simulink model "Quadcopter_nonlinear"  (R2020a)
settings: Solver=ode4  StartTime=0.0  StopTime=0.5  FixedStep=0.02  RelTol=1e-3
InitFcn:
  | QuadParameter
values from neighbouring files (symbols this model uses):
  d = 3.2e-6    (= 3.2e-06)    [QuadParameter.m]    (also in Scenario_III.mat)
  g = 9.81    [QuadParameter.m]
  init_I = data(1, :)    [load_data.m]
  init_II = data(1, :)    [load_data.m]
  init_III = data(1, :)    [load_data.m]
  init_IV = data(1, :)    [load_data.m]
  init_V = data(1, :)    [load_data.m]
  J_zz = 0.058510    (= 0.05851)    [QuadParameter.m]
  m3 = 1.693    [QuadParameter.m]
  miu_k = 0.002    [QuadParameter.m]
  Omega_I = Omega_data    [load_data.m]
  Omega_II = Omega_data    [load_data.m]
  Omega_III = Omega_data    [load_data.m]
  Omega_IV = Omega_data    [load_data.m]
  Omega_V = Omega_data    [load_data.m]
  r_z = 0.025    [QuadParameter.m]
undefined symbols (not defined in the file or in its folder): magnitude
settings Model: OrderedModelArguments=off  Creator=Ali  LastModifiedBy=Ali

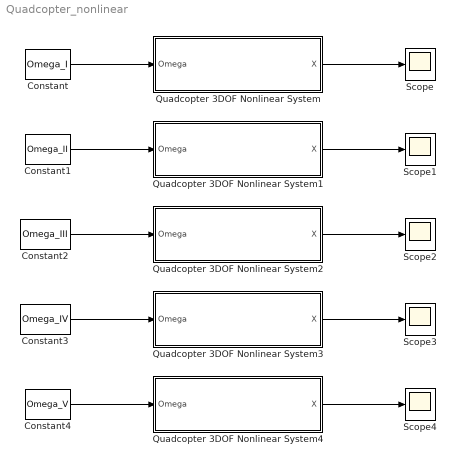
== system Quadcopter_nonlinear ==
  Constant : Constant  Value=Omega_I
  Constant1 : Constant  Value=Omega_II
  Constant2 : Constant  Value=Omega_III
  Constant3 : Constant  Value=Omega_IV
  Constant4 : Constant  Value=Omega_V
  Quadcopter 3DOF Nonlinear System : Subsystem  TreatAsAtomicUnit=on
  Quadcopter 3DOF Nonlinear System1 : Subsystem  TreatAsAtomicUnit=on
  Quadcopter 3DOF Nonlinear System2 : Subsystem  TreatAsAtomicUnit=on
  Quadcopter 3DOF Nonlinear System3 : Subsystem  TreatAsAtomicUnit=on
  Quadcopter 3DOF Nonlinear System4 : Subsystem  TreatAsAtomicUnit=on
  Scope{,1..4} (5 alike) : Scope
  wires:
  Quadcopter 3DOF Nonlinear System/1(X) -> Scope/1
  Constant/1 -> Quadcopter 3DOF Nonlinear System/1(Omega)
  Constant1/1 -> Quadcopter 3DOF Nonlinear System1/1(Omega)
  Quadcopter 3DOF Nonlinear System1/1(X) -> Scope1/1
  Constant2/1 -> Quadcopter 3DOF Nonlinear System2/1(Omega)
  Quadcopter 3DOF Nonlinear System2/1(X) -> Scope2/1
  Constant3/1 -> Quadcopter 3DOF Nonlinear System3/1(Omega)
  Quadcopter 3DOF Nonlinear System3/1(X) -> Scope3/1
  Constant4/1 -> Quadcopter 3DOF Nonlinear System4/1(Omega)
  Quadcopter 3DOF Nonlinear System4/1(X) -> Scope4/1

== system Quadcopter_nonlinear/Quadcopter 3DOF Nonlinear System ==
  Omega : Inport
  Integrator : Integrator  InitialCondition=init_I
  Quad System : Subsystem
  X : Outport
  wires:
  Integrator/1 -> Quad System/1(X), X/1  "X"
  Quad System/1(dot(X)) -> Integrator/1  "dot(X)"
  Omega/1 -> Quad System/2(Omega)

== system Quadcopter_nonlinear/Quadcopter 3DOF Nonlinear System1 ==
  Omega : Inport
  Integrator : Integrator  InitialCondition=init_II
  Quad System : Subsystem
  X : Outport
  wires:
  Integrator/1 -> Quad System/1(X), X/1  "X"
  Quad System/1(dot(X)) -> Integrator/1  "dot(X)"
  Omega/1 -> Quad System/2(Omega)

== system Quadcopter_nonlinear/Quadcopter 3DOF Nonlinear System2 ==
  Omega : Inport
  Integrator : Integrator  InitialCondition=init_III
  Quad System : Subsystem
  X : Outport
  wires:
  Integrator/1 -> Quad System/1(X), X/1  "X"
  Quad System/1(dot(X)) -> Integrator/1  "dot(X)"
  Omega/1 -> Quad System/2(Omega)

== system Quadcopter_nonlinear/Quadcopter 3DOF Nonlinear System3 ==
  Omega : Inport
  Integrator : Integrator  InitialCondition=init_IV
  Quad System : Subsystem
  X : Outport
  wires:
  Integrator/1 -> Quad System/1(X), X/1  "X"
  Quad System/1(dot(X)) -> Integrator/1  "dot(X)"
  Omega/1 -> Quad System/2(Omega)

== system Quadcopter_nonlinear/Quadcopter 3DOF Nonlinear System4 ==
  Omega : Inport
  Integrator : Integrator  InitialCondition=init_V
  Quad System : Subsystem
  X : Outport
  wires:
  Integrator/1 -> Quad System/1(X), X/1  "X"
  Quad System/1(dot(X)) -> Integrator/1  "dot(X)"
  Omega/1 -> Quad System/2(Omega)

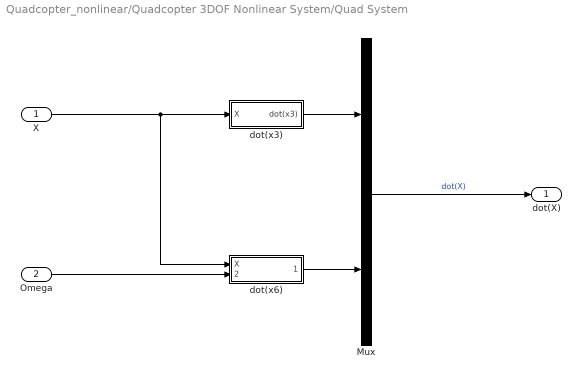
== system Quadcopter_nonlinear/Quadcopter 3DOF Nonlinear System/Quad System ==
  X : Inport
  Omega : Inport  Port=2
  Mux : Mux  Inputs=2
  dot(x3) : Subsystem
  dot(x6) : Subsystem
  dot(X) : Outport
  wires:
  Mux/1 -> dot(X)/1  "dot(X)"
  X/1 -> dot(x6)/1(X), dot(x3)/1(X)
  Omega/1 -> dot(x6)/2(Omega)
  dot(x3)/1(dot(x3)) -> Mux/1
  dot(x6)/1(dot(x6)) -> Mux/2

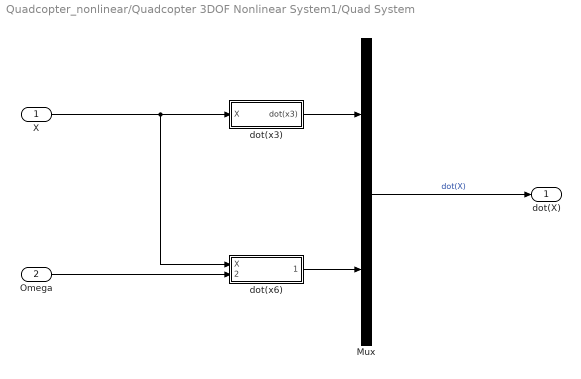
== system Quadcopter_nonlinear/Quadcopter 3DOF Nonlinear System1/Quad System ==
  X : Inport
  Omega : Inport  Port=2
  Mux : Mux  Inputs=2
  dot(x3) : Subsystem
  dot(x6) : Subsystem
  dot(X) : Outport
  wires:
  Mux/1 -> dot(X)/1  "dot(X)"
  X/1 -> dot(x6)/1(X), dot(x3)/1(X)
  Omega/1 -> dot(x6)/2(Omega)
  dot(x3)/1(dot(x3)) -> Mux/1
  dot(x6)/1(dot(x6)) -> Mux/2

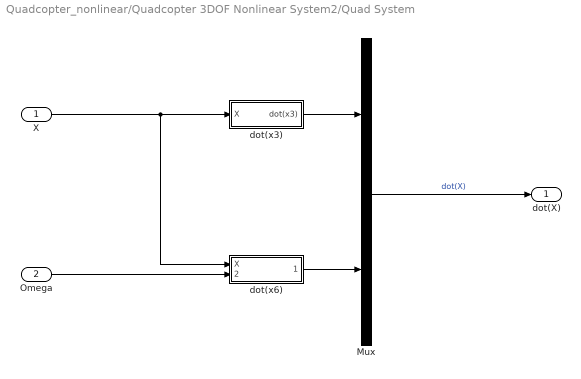
== system Quadcopter_nonlinear/Quadcopter 3DOF Nonlinear System2/Quad System ==
  X : Inport
  Omega : Inport  Port=2
  Mux : Mux  Inputs=2
  dot(x3) : Subsystem
  dot(x6) : Subsystem
  dot(X) : Outport
  wires:
  Mux/1 -> dot(X)/1  "dot(X)"
  X/1 -> dot(x6)/1(X), dot(x3)/1(X)
  Omega/1 -> dot(x6)/2(Omega)
  dot(x3)/1(dot(x3)) -> Mux/1
  dot(x6)/1(dot(x6)) -> Mux/2

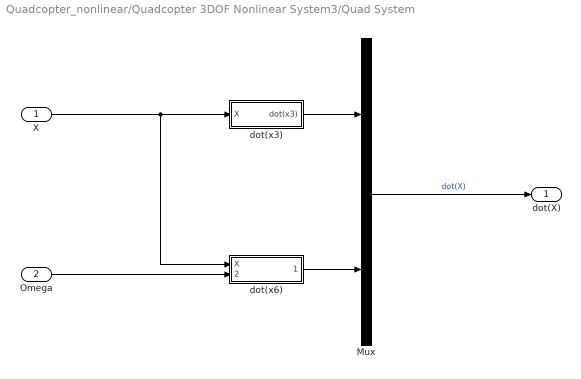
== system Quadcopter_nonlinear/Quadcopter 3DOF Nonlinear System3/Quad System ==
  X : Inport
  Omega : Inport  Port=2
  Mux : Mux  Inputs=2
  dot(x3) : Subsystem
  dot(x6) : Subsystem
  dot(X) : Outport
  wires:
  Mux/1 -> dot(X)/1  "dot(X)"
  X/1 -> dot(x6)/1(X), dot(x3)/1(X)
  Omega/1 -> dot(x6)/2(Omega)
  dot(x3)/1(dot(x3)) -> Mux/1
  dot(x6)/1(dot(x6)) -> Mux/2

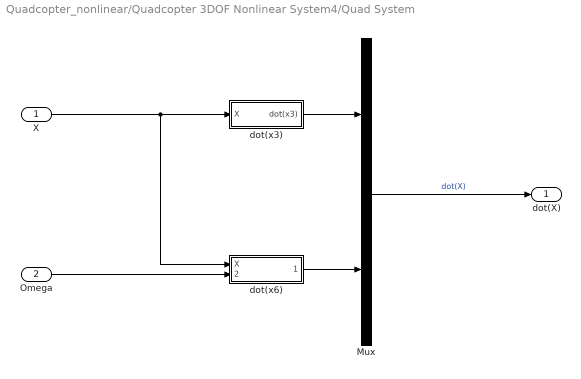
== system Quadcopter_nonlinear/Quadcopter 3DOF Nonlinear System4/Quad System ==
  X : Inport
  Omega : Inport  Port=2
  Mux : Mux  Inputs=2
  dot(x3) : Subsystem
  dot(x6) : Subsystem
  dot(X) : Outport
  wires:
  Mux/1 -> dot(X)/1  "dot(X)"
  X/1 -> dot(x6)/1(X), dot(x3)/1(X)
  Omega/1 -> dot(x6)/2(Omega)
  dot(x3)/1(dot(x3)) -> Mux/1
  dot(x6)/1(dot(x6)) -> Mux/2

== system Quadcopter_nonlinear/Quadcopter 3DOF Nonlinear System/Quad System/dot(x3) ==
  X : Inport
  Subsystem : Subsystem
  dot(x3) : Outport
  wires:
  X/1 -> Subsystem/1(X)  "X"
  Subsystem/1(x6cos(x1)) -> dot(x3)/1

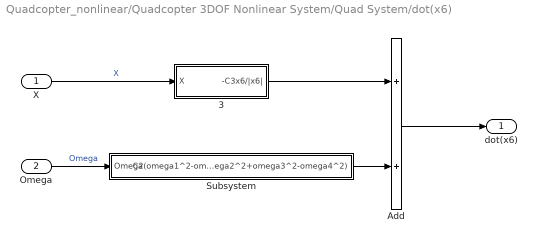
== system Quadcopter_nonlinear/Quadcopter 3DOF Nonlinear System/Quad System/dot(x6) ==
  X : Inport
  Omega : Inport  Port=2
  3 : Subsystem
  Add : Sum
  Subsystem : Subsystem
  dot(x6) : Outport
  wires:
  Omega/1 -> Subsystem/1(Omega)  "Omega"
  Add/1 -> dot(x6)/1
  3/1("-C3x6/|x6| ") -> Add/1
  Subsystem/1(C2(omega1^2-omega2^2+omega3^2-omega4^2)) -> Add/2
  X/1 -> 3/1(X)  "X"

== system Quadcopter_nonlinear/Quadcopter 3DOF Nonlinear System1/Quad System/dot(x3) ==
  X : Inport
  Subsystem : Subsystem
  dot(x3) : Outport
  wires:
  X/1 -> Subsystem/1(X)  "X"
  Subsystem/1(x6cos(x1)) -> dot(x3)/1

== system Quadcopter_nonlinear/Quadcopter 3DOF Nonlinear System1/Quad System/dot(x6) ==
  X : Inport
  Omega : Inport  Port=2
  3 : Subsystem
  Add : Sum
  Subsystem : Subsystem
  dot(x6) : Outport
  wires:
  Omega/1 -> Subsystem/1(Omega)  "Omega"
  Add/1 -> dot(x6)/1
  3/1("-C3x6/|x6| ") -> Add/1
  Subsystem/1(C2(omega1^2-omega2^2+omega3^2-omega4^2)) -> Add/2
  X/1 -> 3/1(X)  "X"

== system Quadcopter_nonlinear/Quadcopter 3DOF Nonlinear System2/Quad System/dot(x3) ==
  X : Inport
  Subsystem : Subsystem
  dot(x3) : Outport
  wires:
  X/1 -> Subsystem/1(X)  "X"
  Subsystem/1(x6cos(x1)) -> dot(x3)/1

== system Quadcopter_nonlinear/Quadcopter 3DOF Nonlinear System2/Quad System/dot(x6) ==
  X : Inport
  Omega : Inport  Port=2
  3 : Subsystem
  Add : Sum
  Subsystem : Subsystem
  dot(x6) : Outport
  wires:
  Omega/1 -> Subsystem/1(Omega)  "Omega"
  Add/1 -> dot(x6)/1
  3/1("-C3x6/|x6| ") -> Add/1
  Subsystem/1(C2(omega1^2-omega2^2+omega3^2-omega4^2)) -> Add/2
  X/1 -> 3/1(X)  "X"

== system Quadcopter_nonlinear/Quadcopter 3DOF Nonlinear System3/Quad System/dot(x3) ==
  X : Inport
  Subsystem : Subsystem
  dot(x3) : Outport
  wires:
  X/1 -> Subsystem/1(X)  "X"
  Subsystem/1(x6cos(x1)) -> dot(x3)/1

== system Quadcopter_nonlinear/Quadcopter 3DOF Nonlinear System3/Quad System/dot(x6) ==
  X : Inport
  Omega : Inport  Port=2
  3 : Subsystem
  Add : Sum
  Subsystem : Subsystem
  dot(x6) : Outport
  wires:
  Omega/1 -> Subsystem/1(Omega)  "Omega"
  Add/1 -> dot(x6)/1
  3/1("-C3x6/|x6| ") -> Add/1
  Subsystem/1(C2(omega1^2-omega2^2+omega3^2-omega4^2)) -> Add/2
  X/1 -> 3/1(X)  "X"

== system Quadcopter_nonlinear/Quadcopter 3DOF Nonlinear System4/Quad System/dot(x3) ==
  X : Inport
  Subsystem : Subsystem
  dot(x3) : Outport
  wires:
  X/1 -> Subsystem/1(X)  "X"
  Subsystem/1(x6cos(x1)) -> dot(x3)/1

== system Quadcopter_nonlinear/Quadcopter 3DOF Nonlinear System4/Quad System/dot(x6) ==
  X : Inport
  Omega : Inport  Port=2
  3 : Subsystem
  Add : Sum
  Subsystem : Subsystem
  dot(x6) : Outport
  wires:
  Omega/1 -> Subsystem/1(Omega)  "Omega"
  Add/1 -> dot(x6)/1
  3/1("-C3x6/|x6| ") -> Add/1
  Subsystem/1(C2(omega1^2-omega2^2+omega3^2-omega4^2)) -> Add/2
  X/1 -> 3/1(X)  "X"

== system Quadcopter_nonlinear/Quadcopter 3DOF Nonlinear System/Quad System/dot(x3)/Subsystem ==
  X : Inport
  Selector : Selector  InputPortWidth=2  IndexOptions=Index vector (dialog)  Indices=[2]  OutputSizes=1
  Subsystem1 : Subsystem
  x6cos(x1) : Outport
  wires:
  Selector/1 -> Subsystem1/1(x6)  "x6"
  Subsystem1/1(Out1) -> x6cos(x1)/1  "x6cos(x1)"
  X/1 -> Selector/1  "X"

== system Quadcopter_nonlinear/Quadcopter 3DOF Nonlinear System/Quad System/dot(x6)/3 ==
  X : Inport
  Selector : Selector  InputPortWidth=2  IndexOptions=Index vector (dialog)  Indices=[2]  OutputSizes=1
  Subsystem : Subsystem
  "-C3x6/|x6| " : Outport
  wires:
  Selector/1 -> Subsystem/1(x6)  "x6"
  Subsystem/1("-C3x6/|x6| ") -> "-C3x6/|x6| "/1
  X/1 -> Selector/1  "x"

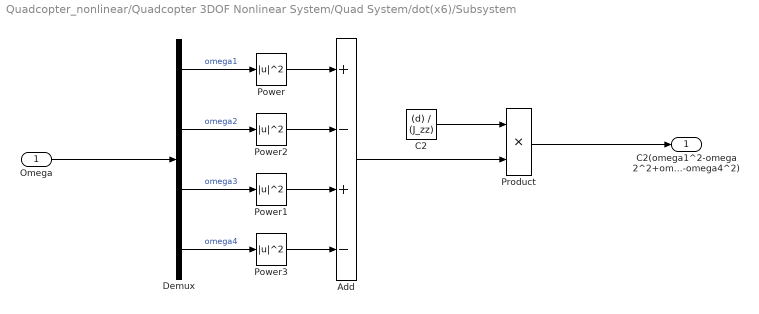
== system Quadcopter_nonlinear/Quadcopter 3DOF Nonlinear System/Quad System/dot(x6)/Subsystem ==
  Omega : Inport
  Add : Sum  Inputs=+-+-
  C2 : Constant  Value=(d) / (J_zz)
  Demux : Demux
  Power{,1..3} (4 alike) : Math  Operator=magnitude^2  SaturateOnIntegerOverflow=on
  Product : Product
  C2(omega1^2-omega2^2+omega3^2-omega4^2) : Outport
  wires:
  Omega/1 -> Demux/1
  Demux/3 -> Power1/1  "omega3"
  Demux/1 -> Power/1  "omega1"
  Demux/2 -> Power2/1  "omega2"
  Demux/4 -> Power3/1  "omega4"
  C2/1 -> Product/1
  Add/1 -> Product/2
  Product/1 -> C2(omega1^2-omega2^2+omega3^2-omega4^2)/1
  Power/1 -> Add/1
  Power2/1 -> Add/2
  Power1/1 -> Add/3
  Power3/1 -> Add/4

== system Quadcopter_nonlinear/Quadcopter 3DOF Nonlinear System1/Quad System/dot(x3)/Subsystem ==
  X : Inport
  Selector : Selector  InputPortWidth=2  IndexOptions=Index vector (dialog)  Indices=[2]  OutputSizes=1
  Subsystem1 : Subsystem
  x6cos(x1) : Outport
  wires:
  Selector/1 -> Subsystem1/1(x6)  "x6"
  Subsystem1/1(Out1) -> x6cos(x1)/1  "x6cos(x1)"
  X/1 -> Selector/1  "X"

== system Quadcopter_nonlinear/Quadcopter 3DOF Nonlinear System1/Quad System/dot(x6)/3 ==
  X : Inport
  Selector : Selector  InputPortWidth=2  IndexOptions=Index vector (dialog)  Indices=[2]  OutputSizes=1
  Subsystem : Subsystem
  "-C3x6/|x6| " : Outport
  wires:
  Selector/1 -> Subsystem/1(x6)  "x6"
  Subsystem/1("-C3x6/|x6| ") -> "-C3x6/|x6| "/1
  X/1 -> Selector/1  "x"

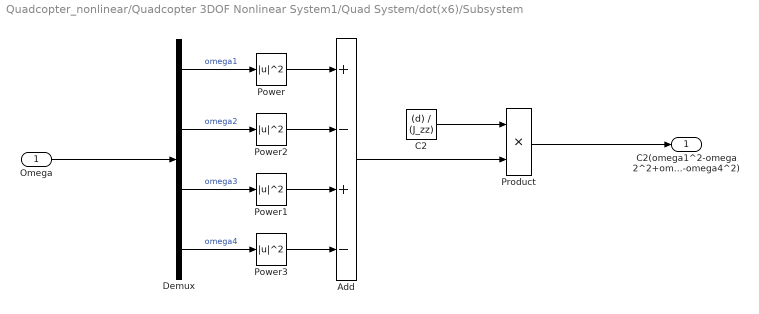
== system Quadcopter_nonlinear/Quadcopter 3DOF Nonlinear System1/Quad System/dot(x6)/Subsystem ==
  Omega : Inport
  Add : Sum  Inputs=+-+-
  C2 : Constant  Value=(d) / (J_zz)
  Demux : Demux
  Power{,1..3} (4 alike) : Math  Operator=magnitude^2  SaturateOnIntegerOverflow=on
  Product : Product
  C2(omega1^2-omega2^2+omega3^2-omega4^2) : Outport
  wires:
  Omega/1 -> Demux/1
  Demux/3 -> Power1/1  "omega3"
  Demux/1 -> Power/1  "omega1"
  Demux/2 -> Power2/1  "omega2"
  Demux/4 -> Power3/1  "omega4"
  C2/1 -> Product/1
  Add/1 -> Product/2
  Product/1 -> C2(omega1^2-omega2^2+omega3^2-omega4^2)/1
  Power/1 -> Add/1
  Power2/1 -> Add/2
  Power1/1 -> Add/3
  Power3/1 -> Add/4

== system Quadcopter_nonlinear/Quadcopter 3DOF Nonlinear System2/Quad System/dot(x3)/Subsystem ==
  X : Inport
  Selector : Selector  InputPortWidth=2  IndexOptions=Index vector (dialog)  Indices=[2]  OutputSizes=1
  Subsystem1 : Subsystem
  x6cos(x1) : Outport
  wires:
  Selector/1 -> Subsystem1/1(x6)  "x6"
  Subsystem1/1(Out1) -> x6cos(x1)/1  "x6cos(x1)"
  X/1 -> Selector/1  "X"

== system Quadcopter_nonlinear/Quadcopter 3DOF Nonlinear System2/Quad System/dot(x6)/3 ==
  X : Inport
  Selector : Selector  InputPortWidth=2  IndexOptions=Index vector (dialog)  Indices=[2]  OutputSizes=1
  Subsystem : Subsystem
  "-C3x6/|x6| " : Outport
  wires:
  Selector/1 -> Subsystem/1(x6)  "x6"
  Subsystem/1("-C3x6/|x6| ") -> "-C3x6/|x6| "/1
  X/1 -> Selector/1  "x"

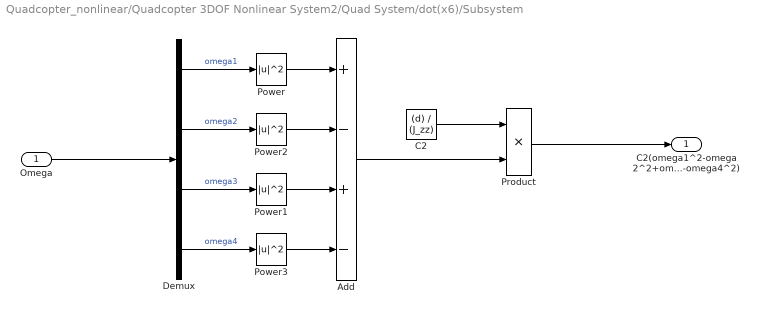
== system Quadcopter_nonlinear/Quadcopter 3DOF Nonlinear System2/Quad System/dot(x6)/Subsystem ==
  Omega : Inport
  Add : Sum  Inputs=+-+-
  C2 : Constant  Value=(d) / (J_zz)
  Demux : Demux
  Power{,1..3} (4 alike) : Math  Operator=magnitude^2  SaturateOnIntegerOverflow=on
  Product : Product
  C2(omega1^2-omega2^2+omega3^2-omega4^2) : Outport
  wires:
  Omega/1 -> Demux/1
  Demux/3 -> Power1/1  "omega3"
  Demux/1 -> Power/1  "omega1"
  Demux/2 -> Power2/1  "omega2"
  Demux/4 -> Power3/1  "omega4"
  C2/1 -> Product/1
  Add/1 -> Product/2
  Product/1 -> C2(omega1^2-omega2^2+omega3^2-omega4^2)/1
  Power/1 -> Add/1
  Power2/1 -> Add/2
  Power1/1 -> Add/3
  Power3/1 -> Add/4

== system Quadcopter_nonlinear/Quadcopter 3DOF Nonlinear System3/Quad System/dot(x3)/Subsystem ==
  X : Inport
  Selector : Selector  InputPortWidth=2  IndexOptions=Index vector (dialog)  Indices=[2]  OutputSizes=1
  Subsystem1 : Subsystem
  x6cos(x1) : Outport
  wires:
  Selector/1 -> Subsystem1/1(x6)  "x6"
  Subsystem1/1(Out1) -> x6cos(x1)/1  "x6cos(x1)"
  X/1 -> Selector/1  "X"

== system Quadcopter_nonlinear/Quadcopter 3DOF Nonlinear System3/Quad System/dot(x6)/3 ==
  X : Inport
  Selector : Selector  InputPortWidth=2  IndexOptions=Index vector (dialog)  Indices=[2]  OutputSizes=1
  Subsystem : Subsystem
  "-C3x6/|x6| " : Outport
  wires:
  Selector/1 -> Subsystem/1(x6)  "x6"
  Subsystem/1("-C3x6/|x6| ") -> "-C3x6/|x6| "/1
  X/1 -> Selector/1  "x"

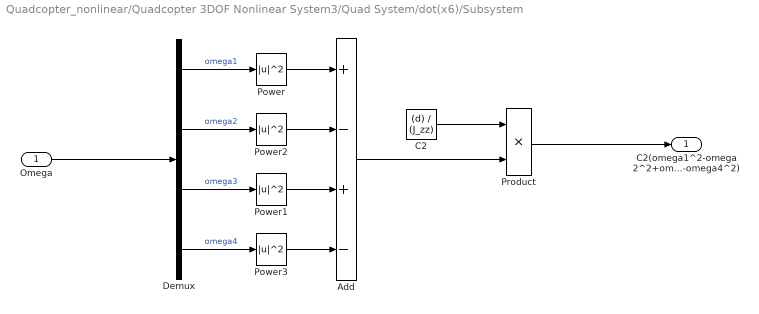
== system Quadcopter_nonlinear/Quadcopter 3DOF Nonlinear System3/Quad System/dot(x6)/Subsystem ==
  Omega : Inport
  Add : Sum  Inputs=+-+-
  C2 : Constant  Value=(d) / (J_zz)
  Demux : Demux
  Power{,1..3} (4 alike) : Math  Operator=magnitude^2  SaturateOnIntegerOverflow=on
  Product : Product
  C2(omega1^2-omega2^2+omega3^2-omega4^2) : Outport
  wires:
  Omega/1 -> Demux/1
  Demux/3 -> Power1/1  "omega3"
  Demux/1 -> Power/1  "omega1"
  Demux/2 -> Power2/1  "omega2"
  Demux/4 -> Power3/1  "omega4"
  C2/1 -> Product/1
  Add/1 -> Product/2
  Product/1 -> C2(omega1^2-omega2^2+omega3^2-omega4^2)/1
  Power/1 -> Add/1
  Power2/1 -> Add/2
  Power1/1 -> Add/3
  Power3/1 -> Add/4

== system Quadcopter_nonlinear/Quadcopter 3DOF Nonlinear System4/Quad System/dot(x3)/Subsystem ==
  X : Inport
  Selector : Selector  InputPortWidth=2  IndexOptions=Index vector (dialog)  Indices=[2]  OutputSizes=1
  Subsystem1 : Subsystem
  x6cos(x1) : Outport
  wires:
  Selector/1 -> Subsystem1/1(x6)  "x6"
  Subsystem1/1(Out1) -> x6cos(x1)/1  "x6cos(x1)"
  X/1 -> Selector/1  "X"

== system Quadcopter_nonlinear/Quadcopter 3DOF Nonlinear System4/Quad System/dot(x6)/3 ==
  X : Inport
  Selector : Selector  InputPortWidth=2  IndexOptions=Index vector (dialog)  Indices=[2]  OutputSizes=1
  Subsystem : Subsystem
  "-C3x6/|x6| " : Outport
  wires:
  Selector/1 -> Subsystem/1(x6)  "x6"
  Subsystem/1("-C3x6/|x6| ") -> "-C3x6/|x6| "/1
  X/1 -> Selector/1  "x"

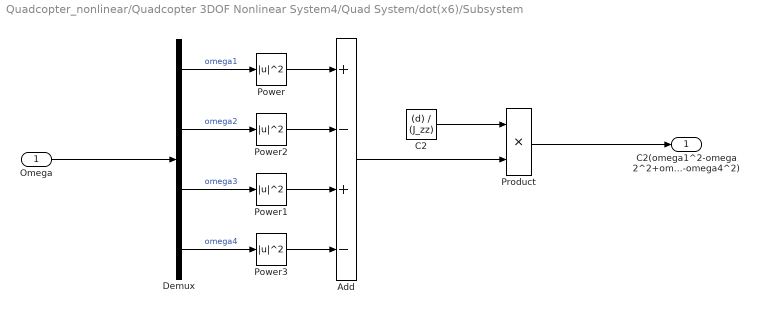
== system Quadcopter_nonlinear/Quadcopter 3DOF Nonlinear System4/Quad System/dot(x6)/Subsystem ==
  Omega : Inport
  Add : Sum  Inputs=+-+-
  C2 : Constant  Value=(d) / (J_zz)
  Demux : Demux
  Power{,1..3} (4 alike) : Math  Operator=magnitude^2  SaturateOnIntegerOverflow=on
  Product : Product
  C2(omega1^2-omega2^2+omega3^2-omega4^2) : Outport
  wires:
  Omega/1 -> Demux/1
  Demux/3 -> Power1/1  "omega3"
  Demux/1 -> Power/1  "omega1"
  Demux/2 -> Power2/1  "omega2"
  Demux/4 -> Power3/1  "omega4"
  C2/1 -> Product/1
  Add/1 -> Product/2
  Product/1 -> C2(omega1^2-omega2^2+omega3^2-omega4^2)/1
  Power/1 -> Add/1
  Power2/1 -> Add/2
  Power1/1 -> Add/3
  Power3/1 -> Add/4

== system Quadcopter_nonlinear/Quadcopter 3DOF Nonlinear System/Quad System/dot(x3)/Subsystem/Subsystem1 ==
  x6 : Inport
  Out1 : Outport
  wires:
  x6/1 -> Out1/1

== system Quadcopter_nonlinear/Quadcopter 3DOF Nonlinear System/Quad System/dot(x6)/3/Subsystem ==
  x6 : Inport
  C3 : Constant  Value=(m3 * g * miu_k * r_z) / (J_zz)
  Gain : Gain  Gain=-1
  Switch : Switch  Criteria=u2 > Threshold
  "-C3x6/|x6| " : Outport
  wires:
  Switch/1 -> "-C3x6/|x6| "/1
  C3/1 -> Switch/3, Gain/1
  x6/1 -> Switch/2
  Gain/1 -> Switch/1

== system Quadcopter_nonlinear/Quadcopter 3DOF Nonlinear System1/Quad System/dot(x3)/Subsystem/Subsystem1 ==
  x6 : Inport
  Out1 : Outport
  wires:
  x6/1 -> Out1/1

== system Quadcopter_nonlinear/Quadcopter 3DOF Nonlinear System1/Quad System/dot(x6)/3/Subsystem ==
  x6 : Inport
  C3 : Constant  Value=(m3 * g * miu_k * r_z) / (J_zz)
  Gain : Gain  Gain=-1
  Switch : Switch  Criteria=u2 > Threshold
  "-C3x6/|x6| " : Outport
  wires:
  Switch/1 -> "-C3x6/|x6| "/1
  C3/1 -> Switch/3, Gain/1
  x6/1 -> Switch/2
  Gain/1 -> Switch/1

== system Quadcopter_nonlinear/Quadcopter 3DOF Nonlinear System2/Quad System/dot(x3)/Subsystem/Subsystem1 ==
  x6 : Inport
  Out1 : Outport
  wires:
  x6/1 -> Out1/1

== system Quadcopter_nonlinear/Quadcopter 3DOF Nonlinear System2/Quad System/dot(x6)/3/Subsystem ==
  x6 : Inport
  C3 : Constant  Value=(m3 * g * miu_k * r_z) / (J_zz)
  Gain : Gain  Gain=-1
  Switch : Switch  Criteria=u2 > Threshold
  "-C3x6/|x6| " : Outport
  wires:
  Switch/1 -> "-C3x6/|x6| "/1
  C3/1 -> Switch/3, Gain/1
  x6/1 -> Switch/2
  Gain/1 -> Switch/1

== system Quadcopter_nonlinear/Quadcopter 3DOF Nonlinear System3/Quad System/dot(x3)/Subsystem/Subsystem1 ==
  x6 : Inport
  Out1 : Outport
  wires:
  x6/1 -> Out1/1

== system Quadcopter_nonlinear/Quadcopter 3DOF Nonlinear System3/Quad System/dot(x6)/3/Subsystem ==
  x6 : Inport
  C3 : Constant  Value=(m3 * g * miu_k * r_z) / (J_zz)
  Gain : Gain  Gain=-1
  Switch : Switch  Criteria=u2 > Threshold
  "-C3x6/|x6| " : Outport
  wires:
  Switch/1 -> "-C3x6/|x6| "/1
  C3/1 -> Switch/3, Gain/1
  x6/1 -> Switch/2
  Gain/1 -> Switch/1

== system Quadcopter_nonlinear/Quadcopter 3DOF Nonlinear System4/Quad System/dot(x3)/Subsystem/Subsystem1 ==
  x6 : Inport
  Out1 : Outport
  wires:
  x6/1 -> Out1/1

== system Quadcopter_nonlinear/Quadcopter 3DOF Nonlinear System4/Quad System/dot(x6)/3/Subsystem ==
  x6 : Inport
  C3 : Constant  Value=(m3 * g * miu_k * r_z) / (J_zz)
  Gain : Gain  Gain=-1
  Switch : Switch  Criteria=u2 > Threshold
  "-C3x6/|x6| " : Outport
  wires:
  Switch/1 -> "-C3x6/|x6| "/1
  C3/1 -> Switch/3, Gain/1
  x6/1 -> Switch/2
  Gain/1 -> Switch/1
